simulink model "gm_IP_Core_SS_Switch_and_PWM"  (R2021a)
settings: Solver=VariableStepAuto  StartTime=0.0  StopTime=0.0002  RelTol=1e-3
undefined symbols (not defined in the file or in its folder): f_FPGA_clk, T_FPGA_clk
libraries: hdlmdlgenlib x3, hdlsllib x3
(part 2 of 2)

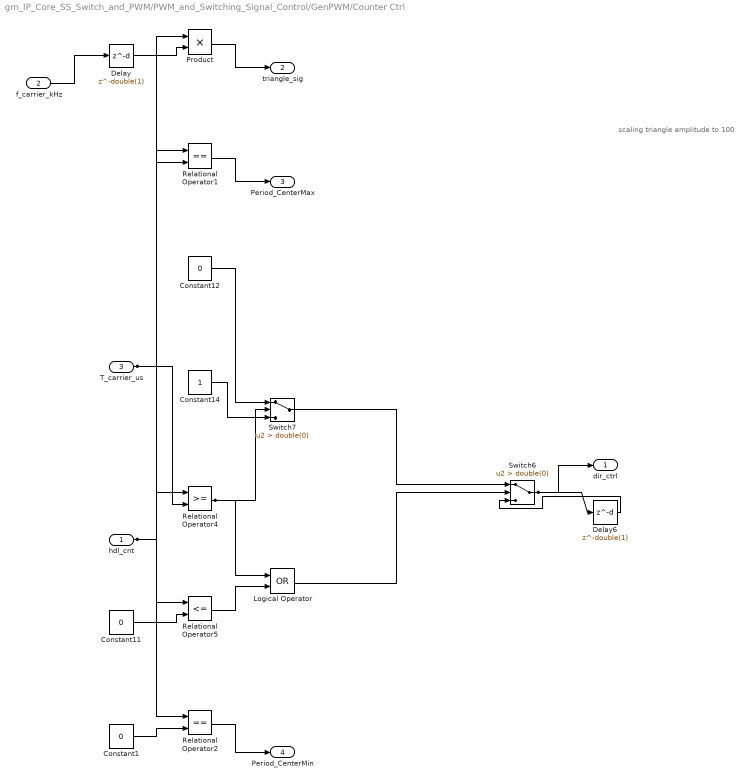
== system gm_IP_Core_SS_Switch_and_PWM/PWM_and_Switching_Signal_Control/GenPWM/Counter Ctrl ==
  note: scaling triangle amplitude to 100
  hdl_cnt : Inport  OutDataTypeStr=fixdt(0, 20, 0)  PortDimensions=1  SampleTime=1e-08
  f_carrier_kHz : Inport  Port=2  OutDataTypeStr=fixdt(0, 25, 26)  PortDimensions=1  SampleTime=1e-08
  T_carrier_us : Inport  Port=3  OutDataTypeStr=fixdt(0, 25, 0)  PortDimensions=1  SampleTime=1e-08
  Constant1 : Constant  Value=0  OutDataTypeStr=fixdt(0, 20, 0)  SampleTime=1e-08
  Constant11 : Constant  Value=0  OutDataTypeStr=fixdt(0, 20, 0)  SampleTime=1e-08
  Constant12 : Constant  Value=0  OutDataTypeStr=boolean  SampleTime=1e-08
  Constant14 : Constant  OutDataTypeStr=boolean  SampleTime=1e-08
  Delay : Delay  DelayLength=double(1)  InitialCondition=0  SampleTime=1e-08
  Delay6 : Delay  DelayLength=double(1)  InitialCondition=0  SampleTime=1e-08
  Logical Operator : Logic  Operator=OR  AllPortsSameDT=off  OutDataTypeStr=boolean  SampleTime=1e-08
  Product : Product  Inputs=**  OutDataTypeStr=fixdt(0, 18, 17)  SampleTime=1e-08
  Relational Operator1 : RelationalOperator  Operator===  OutDataTypeStr=boolean  SampleTime=1e-08  RndMeth=Nearest
  Relational Operator2 : RelationalOperator  Operator===  OutDataTypeStr=boolean  SampleTime=1e-08  RndMeth=Nearest
  Relational Operator4 : RelationalOperator  OutDataTypeStr=boolean  SampleTime=1e-08  RndMeth=Nearest
  Relational Operator5 : RelationalOperator  Operator=<=  OutDataTypeStr=boolean  SampleTime=1e-08  RndMeth=Nearest
  Switch6 : Switch  Criteria=u2 > Threshold  Threshold=double(0)  OutDataTypeStr=boolean  SampleTime=1e-08
  Switch7 : Switch  Criteria=u2 > Threshold  Threshold=double(0)  OutDataTypeStr=boolean  SampleTime=1e-08
  dir_ctrl : Outport  SampleTime=1e-08  VectorParamsAs1DForOutWhenUnconnected=off
  triangle_sig : Outport  Port=2  SampleTime=1e-08  VectorParamsAs1DForOutWhenUnconnected=off
  Period_CenterMax : Outport  Port=3  SampleTime=1e-08  VectorParamsAs1DForOutWhenUnconnected=off
  Period_CenterMin : Outport  Port=4  SampleTime=1e-08  VectorParamsAs1DForOutWhenUnconnected=off
  wires:
  hdl_cnt/1 -> Relational Operator5/1, Relational Operator4/1, Relational Operator2/1, Relational Operator1/1, Product/1
  f_carrier_kHz/1 -> Delay/1
  T_carrier_us/1 -> Relational Operator4/2, Relational Operator1/2
  Constant1/1 -> Relational Operator2/2
  Constant11/1 -> Relational Operator5/2
  Constant12/1 -> Switch7/1
  Constant14/1 -> Switch7/3
  Delay/1 -> Product/2
  Delay6/1 -> Switch6/3
  Logical Operator/1 -> Switch6/2
  Product/1 -> triangle_sig/1
  Relational Operator1/1 -> Period_CenterMax/1
  Relational Operator2/1 -> Period_CenterMin/1
  Relational Operator4/1 -> Switch7/2, Logical Operator/1
  Relational Operator5/1 -> Logical Operator/2
  Switch6/1 -> Delay6/1, dir_ctrl/1
  Switch7/1 -> Switch6/1

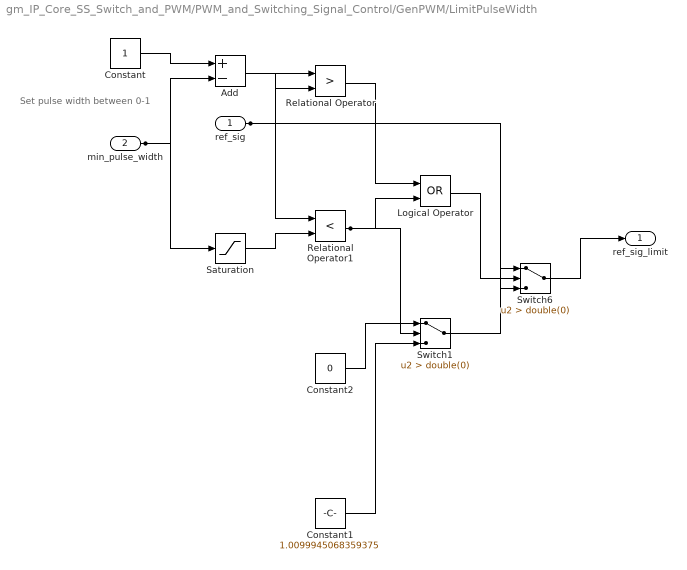
== system gm_IP_Core_SS_Switch_and_PWM/PWM_and_Switching_Signal_Control/GenPWM/LimitPulseWidth ==
  note: Set pulse width between 0-1
  ref_sig : Inport  OutDataTypeStr=fixdt(1, 14, 12)  PortDimensions=1  SampleTime=1e-08
  min_pulse_width : Inport  Port=2  OutDataTypeStr=fixdt(1, 18, 16)  PortDimensions=1  SampleTime=1e-08
  Add : Sum  Inputs=+-  AccumDataTypeStr=fixdt(1, 19, 16)  OutDataTypeStr=fixdt(1, 18, 16)  SampleTime=1e-08
  Constant : Constant  OutDataTypeStr=fixdt(1, 18, 16)  SampleTime=1e-08
  Constant1 : Constant  Value=1.0099945068359375  OutDataTypeStr=fixdt(1, 18, 16)  SampleTime=1e-08
  Constant2 : Constant  Value=0  OutDataTypeStr=fixdt(1, 18, 16)  SampleTime=1e-08
  Logical Operator : Logic  Operator=OR  AllPortsSameDT=off  OutDataTypeStr=boolean  SampleTime=1e-08
  Relational Operator : RelationalOperator  Operator=>  OutDataTypeStr=boolean  SampleTime=1e-08  RndMeth=Nearest
  Relational Operator1 : RelationalOperator  Operator=<  OutDataTypeStr=boolean  SampleTime=1e-08  RndMeth=Nearest
  Saturation : Saturate  UpperLimit="fi(0,1,18,16,\"hex\",\"10000\")"  LowerLimit="fi(0,1,18,16,\"hex\",\"00000\")"  SampleTime=1e-08  OutDataTypeStr=fixdt(1, 18, 16)
  Switch1 : Switch  Criteria=u2 > Threshold  Threshold=double(0)  OutDataTypeStr=fixdt(1, 18, 16)  SampleTime=1e-08
  Switch6 : Switch  Criteria=u2 > Threshold  Threshold=double(0)  OutDataTypeStr=fixdt(1, 18, 16)  SampleTime=1e-08
  ref_sig_limit : Outport  SampleTime=1e-08  VectorParamsAs1DForOutWhenUnconnected=off
  wires:
  Add/1 -> Relational Operator/2
  Constant/1 -> Add/1
  Constant1/1 -> Switch1/3
  Constant2/1 -> Switch1/1
  Logical Operator/1 -> Switch6/2
  Relational Operator/1 -> Logical Operator/1
  Relational Operator1/1 -> Switch1/2, Logical Operator/2
  Saturation/1 -> Relational Operator1/2
  Switch1/1 -> Switch6/1
  Switch6/1 -> ref_sig_limit/1
  ref_sig/1 -> Switch6/3, Relational Operator1/1, Relational Operator/1
  min_pulse_width/1 -> Saturation/1, Add/2

== system gm_IP_Core_SS_Switch_and_PWM/PWM_and_Switching_Signal_Control/GenPWM/LimitPulseWidth1 ==
  note: Set pulse width in percent
  ref_sig : Inport  OutDataTypeStr=fixdt(1, 14, 12)  PortDimensions=1  SampleTime=1e-08
  min_pulse_width : Inport  Port=2  OutDataTypeStr=fixdt(1, 18, 16)  PortDimensions=1  SampleTime=1e-08
  Add : Sum  Inputs=+-  AccumDataTypeStr=fixdt(1, 19, 16)  OutDataTypeStr=fixdt(1, 18, 16)  SampleTime=1e-08
  Constant : Constant  OutDataTypeStr=fixdt(1, 18, 16)  SampleTime=1e-08
  Constant1 : Constant  Value=1.0099945068359375  OutDataTypeStr=fixdt(1, 18, 16)  SampleTime=1e-08
  Constant2 : Constant  Value=0  OutDataTypeStr=fixdt(1, 18, 16)  SampleTime=1e-08
  Logical Operator : Logic  Operator=OR  AllPortsSameDT=off  OutDataTypeStr=boolean  SampleTime=1e-08
  Relational Operator : RelationalOperator  Operator=>  OutDataTypeStr=boolean  SampleTime=1e-08  RndMeth=Nearest
  Relational Operator1 : RelationalOperator  Operator=<  OutDataTypeStr=boolean  SampleTime=1e-08  RndMeth=Nearest
  Saturation : Saturate  UpperLimit="fi(0,1,18,16,\"hex\",\"10000\")"  LowerLimit="fi(0,1,18,16,\"hex\",\"00000\")"  SampleTime=1e-08  OutDataTypeStr=fixdt(1, 18, 16)
  Switch1 : Switch  Criteria=u2 > Threshold  Threshold=double(0)  OutDataTypeStr=fixdt(1, 18, 16)  SampleTime=1e-08
  Switch6 : Switch  Criteria=u2 > Threshold  Threshold=double(0)  OutDataTypeStr=fixdt(1, 18, 16)  SampleTime=1e-08
  ref_sig_limit : Outport  SampleTime=1e-08  VectorParamsAs1DForOutWhenUnconnected=off
  wires:
  Add/1 -> Relational Operator/2
  Constant/1 -> Add/1
  Constant1/1 -> Switch1/3
  Constant2/1 -> Switch1/1
  Logical Operator/1 -> Switch6/2
  Relational Operator/1 -> Logical Operator/1
  Relational Operator1/1 -> Switch1/2, Logical Operator/2
  Saturation/1 -> Relational Operator1/2
  Switch1/1 -> Switch6/1
  Switch6/1 -> ref_sig_limit/1
  ref_sig/1 -> Switch6/3, Relational Operator1/1, Relational Operator/1
  min_pulse_width/1 -> Saturation/1, Add/2

== system gm_IP_Core_SS_Switch_and_PWM/PWM_and_Switching_Signal_Control/GenPWM/LimitPulseWidth2 ==
  note: Set pulse width in percent
  ref_sig : Inport  OutDataTypeStr=fixdt(1, 14, 12)  PortDimensions=1  SampleTime=1e-08
  min_pulse_width : Inport  Port=2  OutDataTypeStr=fixdt(1, 18, 16)  PortDimensions=1  SampleTime=1e-08
  Add : Sum  Inputs=+-  AccumDataTypeStr=fixdt(1, 19, 16)  OutDataTypeStr=fixdt(1, 18, 16)  SampleTime=1e-08
  Constant : Constant  OutDataTypeStr=fixdt(1, 18, 16)  SampleTime=1e-08
  Constant1 : Constant  Value=1.0099945068359375  OutDataTypeStr=fixdt(1, 18, 16)  SampleTime=1e-08
  Constant2 : Constant  Value=0  OutDataTypeStr=fixdt(1, 18, 16)  SampleTime=1e-08
  Logical Operator : Logic  Operator=OR  AllPortsSameDT=off  OutDataTypeStr=boolean  SampleTime=1e-08
  Relational Operator : RelationalOperator  Operator=>  OutDataTypeStr=boolean  SampleTime=1e-08  RndMeth=Nearest
  Relational Operator1 : RelationalOperator  Operator=<  OutDataTypeStr=boolean  SampleTime=1e-08  RndMeth=Nearest
  Saturation : Saturate  UpperLimit="fi(0,1,18,16,\"hex\",\"10000\")"  LowerLimit="fi(0,1,18,16,\"hex\",\"00000\")"  SampleTime=1e-08  OutDataTypeStr=fixdt(1, 18, 16)
  Switch1 : Switch  Criteria=u2 > Threshold  Threshold=double(0)  OutDataTypeStr=fixdt(1, 18, 16)  SampleTime=1e-08
  Switch6 : Switch  Criteria=u2 > Threshold  Threshold=double(0)  OutDataTypeStr=fixdt(1, 18, 16)  SampleTime=1e-08
  ref_sig_limit : Outport  SampleTime=1e-08  VectorParamsAs1DForOutWhenUnconnected=off
  wires:
  Add/1 -> Relational Operator/2
  Constant/1 -> Add/1
  Constant1/1 -> Switch1/3
  Constant2/1 -> Switch1/1
  Logical Operator/1 -> Switch6/2
  Relational Operator/1 -> Logical Operator/1
  Relational Operator1/1 -> Switch1/2, Logical Operator/2
  Saturation/1 -> Relational Operator1/2
  Switch1/1 -> Switch6/1
  Switch6/1 -> ref_sig_limit/1
  ref_sig/1 -> Switch6/3, Relational Operator1/1, Relational Operator/1
  min_pulse_width/1 -> Saturation/1, Add/2

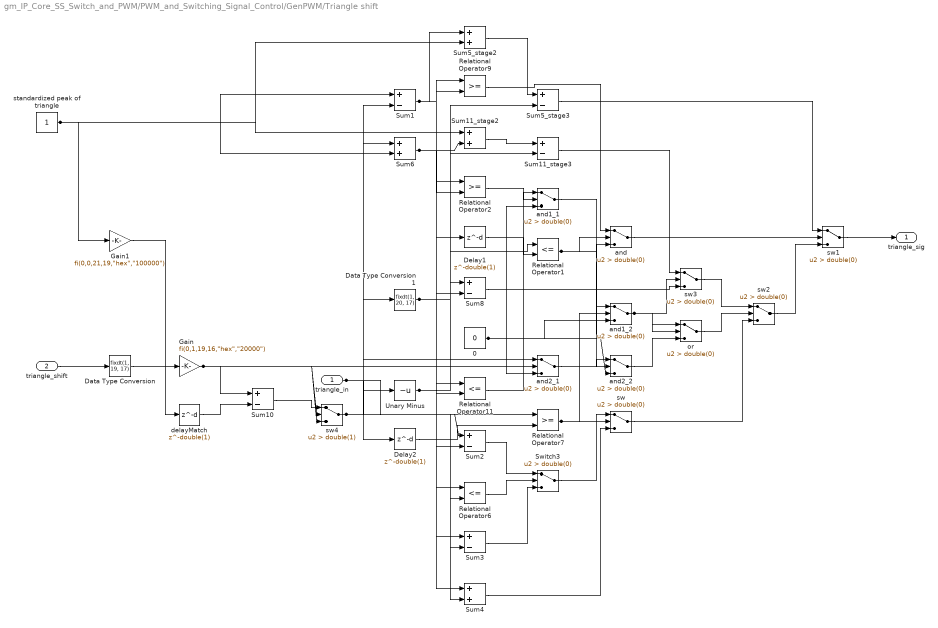
== system gm_IP_Core_SS_Switch_and_PWM/PWM_and_Switching_Signal_Control/GenPWM/Triangle shift ==
  triangle_in : Inport  OutDataTypeStr=fixdt(0, 18, 17)  PortDimensions=1  SampleTime=1e-08
  triangle_shift : Inport  Port=2  OutDataTypeStr=fixdt(0, 18, 17)  PortDimensions=1  SampleTime=1e-08
  0 : Constant  Value=0  OutDataTypeStr=boolean  SampleTime=1e-08
  Data Type Conversion : DataTypeConversion  OutDataTypeStr=fixdt(1, 19, 17)  SampleTime=1e-08
  Data Type Conversion1 : DataTypeConversion  OutDataTypeStr=fixdt(1, 20, 17)  SampleTime=1e-08
  Delay1 : Delay  DelayLength=double(1)  InitialCondition=0  SampleTime=1e-08
  Delay2 : Delay  DelayLength=double(1)  InitialCondition=0  SampleTime=1e-08
  Gain : Gain  Gain="fi(0,1,19,16,\"hex\",\"20000\")"  ParamDataTypeStr=fixdt(1, 19, 16)  OutDataTypeStr=fixdt(1, 20, 17)  SampleTime=1e-08
  Gain1 : Gain  Gain="fi(0,0,21,19,\"hex\",\"100000\")"  ParamDataTypeStr=fixdt(0, 21, 19)  OutDataTypeStr=fixdt(1, 20, 17)  SampleTime=1e-08
  Relational Operator1 : RelationalOperator  Operator=<=  OutDataTypeStr=boolean  SampleTime=1e-08  RndMeth=Nearest
  Relational Operator11 : RelationalOperator  Operator=<=  OutDataTypeStr=boolean  SampleTime=1e-08  RndMeth=Nearest
  Relational Operator2 : RelationalOperator  OutDataTypeStr=boolean  SampleTime=1e-08  RndMeth=Nearest
  Relational Operator6 : RelationalOperator  Operator=<=  OutDataTypeStr=boolean  SampleTime=1e-08  RndMeth=Nearest
  Relational Operator7 : RelationalOperator  OutDataTypeStr=boolean  SampleTime=1e-08  RndMeth=Nearest
  Relational Operator9 : RelationalOperator  OutDataTypeStr=boolean  SampleTime=1e-08  RndMeth=Nearest
  Sum1 : Sum  Inputs=+-  AccumDataTypeStr=fixdt(1, 23, 17)  OutDataTypeStr=fixdt(1, 23, 17)  SampleTime=1e-08
  Sum10 : Sum  Inputs=+-  AccumDataTypeStr=fixdt(1, 21, 17)  OutDataTypeStr=fixdt(1, 20, 17)  SampleTime=1e-08
  Sum11_stage2 : Sum  AccumDataTypeStr=fixdt(1, 24, 17)  OutDataTypeStr=fixdt(1, 24, 17)  SampleTime=1e-08
  Sum11_stage3 : Sum  Inputs=+-  AccumDataTypeStr=fixdt(1, 24, 17)  OutDataTypeStr=fixdt(1, 21, 17)  SampleTime=1e-08
  Sum2 : Sum  Inputs=+-  AccumDataTypeStr=fixdt(1, 21, 17)  OutDataTypeStr=fixdt(1, 21, 17)  SampleTime=1e-08
  Sum3 : Sum  Inputs=+-  AccumDataTypeStr=fixdt(1, 21, 17)  OutDataTypeStr=fixdt(1, 21, 17)  SampleTime=1e-08
  Sum4 : Sum  AccumDataTypeStr=fixdt(1, 21, 17)  OutDataTypeStr=fixdt(1, 21, 17)  SampleTime=1e-08
  Sum5_stage2 : Sum  AccumDataTypeStr=fixdt(1, 24, 17)  OutDataTypeStr=fixdt(1, 24, 17)  SampleTime=1e-08
  Sum5_stage3 : Sum  Inputs=+-  AccumDataTypeStr=fixdt(1, 24, 17)  OutDataTypeStr=fixdt(1, 21, 17)  SampleTime=1e-08
  Sum6 : Sum  AccumDataTypeStr=fixdt(1, 23, 17)  OutDataTypeStr=fixdt(1, 23, 17)  SampleTime=1e-08
  Sum8 : Sum  Inputs=+-  AccumDataTypeStr=fixdt(1, 21, 17)  OutDataTypeStr=fixdt(1, 21, 17)  SampleTime=1e-08
  Switch3 : Switch  Criteria=u2 > Threshold  Threshold=double(0)  OutDataTypeStr=fixdt(1, 21, 17)  SampleTime=1e-08
  Unary Minus : UnaryMinus  SampleTime=1e-08
  and : Switch  Criteria=u2 > Threshold  Threshold=double(0)  OutDataTypeStr=boolean  SampleTime=1e-08
  and1_1 : Switch  Criteria=u2 > Threshold  Threshold=double(0)  OutDataTypeStr=boolean  SampleTime=1e-08
  and1_2 : Switch  Criteria=u2 > Threshold  Threshold=double(0)  OutDataTypeStr=boolean  SampleTime=1e-08
  and2_1 : Switch  Criteria=u2 > Threshold  Threshold=double(0)  OutDataTypeStr=boolean  SampleTime=1e-08
  and2_2 : Switch  Criteria=u2 > Threshold  Threshold=double(0)  OutDataTypeStr=boolean  SampleTime=1e-08
  delayMatch : Delay  DelayLength=double(1)  InitialCondition=0  SampleTime=1e-08
  or : Switch  Criteria=u2 > Threshold  Threshold=double(0)  OutDataTypeStr=boolean  SampleTime=1e-08
  standardized peak of triangle : Constant  OutDataTypeStr=fixdt(0, 21, 17)  SampleTime=1e-08
  sw : Switch  Criteria=u2 > Threshold  Threshold=double(0)  OutDataTypeStr=fixdt(1, 21, 17)  SampleTime=1e-08
  sw1 : Switch  Criteria=u2 > Threshold  Threshold=double(0)  OutDataTypeStr=fixdt(1, 18, 16)  SampleTime=1e-08
  sw2 : Switch  Criteria=u2 > Threshold  Threshold=double(0)  OutDataTypeStr=fixdt(1, 21, 17)  SampleTime=1e-08
  sw3 : Switch  Criteria=u2 > Threshold  Threshold=double(0)  OutDataTypeStr=fixdt(1, 21, 17)  SampleTime=1e-08
  sw4 : Switch  Criteria=u2 > Threshold  Threshold=double(1)  OutDataTypeStr=fixdt(1, 20, 17)  SampleTime=1e-08
  triangle_sig : Outport  SampleTime=1e-08  VectorParamsAs1DForOutWhenUnconnected=off
  wires:
  0/1 -> and2_2/3, and2_1/3, and1_2/3, and1_1/3, and/3
  Data Type Conversion/1 -> Gain/1
  Data Type Conversion1/1 -> Sum8/2, Sum5_stage3/2, Sum4/1, Sum3/1, Sum2/2, Sum11_stage3/2, Relational Operator9/1, Relational Operator6/1, Relational Operator2/1, Relational Operator11/1, Relational Operator1/1, Delay1/1
  Delay1/1 -> Relational Operator1/2
  Delay2/1 -> Relational Operator7/2
  Gain/1 -> sw4/3, sw4/2, and2_1/1, and1_1/1, Sum10/1
  delayMatch/1 -> Sum10/2
  Relational Operator1/1 -> and2_2/2, and/2
  Relational Operator11/1 -> and2_1/2
  Relational Operator2/1 -> and1_1/2
  Relational Operator6/1 -> Switch3/2
  Relational Operator7/1 -> sw/2, and1_2/2
  Relational Operator9/1 -> and/1
  Sum1/1 -> Sum5_stage2/1, Relational Operator9/2
  Sum10/1 -> sw4/1
  Sum11_stage3/1 -> sw3/1
  Sum2/1 -> Switch3/1
  Sum3/1 -> Switch3/3
  Sum4/1 -> sw/3
  Sum5_stage3/1 -> sw1/1
  Sum6/1 -> Sum11_stage2/2, Relational Operator2/2
  Sum8/1 -> sw3/3
  Switch3/1 -> sw/1
  Unary Minus/1 -> Sum8/1, Relational Operator11/2
  and/1 -> sw1/2
  and1_1/1 -> and1_2/1
  and1_2/1 -> sw3/2, or/2, or/1
  and2_1/1 -> and2_2/1
  and2_2/1 -> or/3
  or/1 -> sw2/2
  standardized peak of triangle/1 -> Sum6/2, Sum5_stage2/2, Sum11_stage2/1, Sum1/1, Gain1/1
  sw/1 -> sw2/3
  sw1/1 -> triangle_sig/1
  sw2/1 -> sw1/3
  sw3/1 -> sw2/1
  sw4/1 -> Unary Minus/1, Sum6/1, Sum4/2, Sum3/2, Sum2/1, Sum1/2, Relational Operator6/2
  Sum11_stage2/1 -> Sum11_stage3/1
  Sum5_stage2/1 -> Sum5_stage3/1
  triangle_in/1 -> Relational Operator7/1, Data Type Conversion1/1, Delay2/1
  triangle_shift/1 -> Data Type Conversion/1
  Gain1/1 -> delayMatch/1

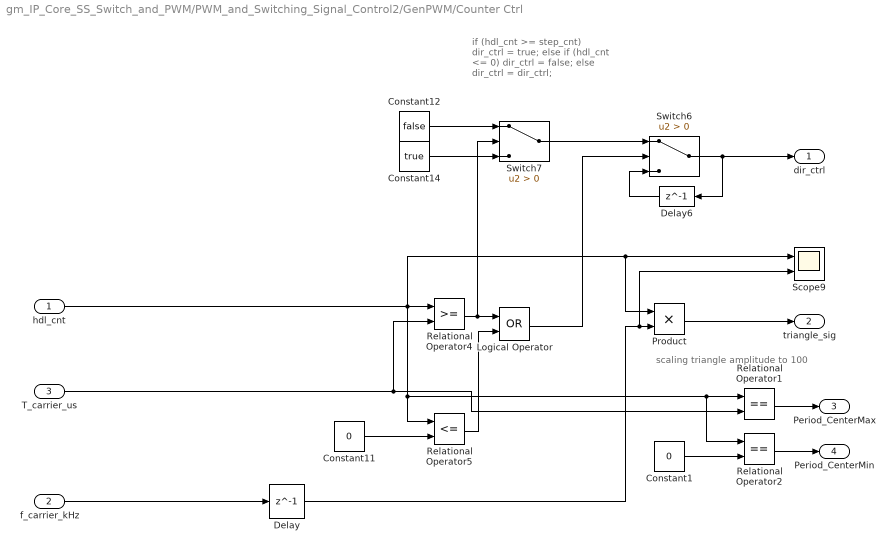
== system gm_IP_Core_SS_Switch_and_PWM/PWM_and_Switching_Signal_Control2/GenPWM/Counter Ctrl ==
  note: scaling triangle amplitude to 100
  note: if (hdl_cnt >= step_cnt)
      | 	dir_ctrl = true;
      | else if (hdl_cnt <= 0)
      | 	dir_ctrl = false;
      | else
      | 	dir_ctrl = dir_ctrl;
  hdl_cnt : Inport
  f_carrier_kHz : Inport  Port=2
  T_carrier_us : Inport  Port=3
  Constant1 : Constant  Value=0  OutDataTypeStr=fixdt(0,20,0)  SampleTime=T_FPGA_clk
  Constant11 : Constant  Value=0  OutDataTypeStr=fixdt(0,20,0)  SampleTime=T_FPGA_clk
  Constant12 : Constant  Value=false  SampleTime=T_FPGA_clk
  Constant14 : Constant  Value=true  SampleTime=T_FPGA_clk
  Delay : Delay  DelayLength=1
  Delay6 : Delay  DelayLength=1
  Logical Operator : Logic  Operator=OR  AllPortsSameDT=off  OutDataTypeStr=boolean
  Product : Product  OutDataTypeStr=fixdt(0,18,17)
  Relational Operator1 : RelationalOperator  Operator===  OutDataTypeStr=boolean  RndMeth=Nearest
  Relational Operator2 : RelationalOperator  Operator===  OutDataTypeStr=boolean  RndMeth=Nearest
  Relational Operator4 : RelationalOperator  OutDataTypeStr=boolean  RndMeth=Nearest
  Relational Operator5 : RelationalOperator  Operator=<=  OutDataTypeStr=boolean  RndMeth=Nearest
  Scope9 : Scope  NumInputPorts=2
  Switch6 : Switch  Criteria=u2 > Threshold
  Switch7 : Switch  Criteria=u2 > Threshold
  dir_ctrl : Outport  VectorParamsAs1DForOutWhenUnconnected=off
  triangle_sig : Outport  Port=2  VectorParamsAs1DForOutWhenUnconnected=off
  Period_CenterMax : Outport  Port=3  VectorParamsAs1DForOutWhenUnconnected=off
  Period_CenterMin : Outport  Port=4  VectorParamsAs1DForOutWhenUnconnected=off
  wires:
  Product/1 -> triangle_sig/1
  Constant1/1 -> Relational Operator2/2
  Relational Operator2/1 -> Period_CenterMin/1
  Relational Operator1/1 -> Period_CenterMax/1
  Delay/1 -> Product/2, Scope9/2
  f_carrier_kHz/1 -> Delay/1
  T_carrier_us/1 -> Relational Operator1/2, Relational Operator4/2
  Delay6/1 -> Switch6/3
  Constant14/1 -> Switch7/3
  Constant12/1 -> Switch7/1
  Switch7/1 -> Switch6/1
  Logical Operator/1 -> Switch6/2
  Constant11/1 -> Relational Operator5/2
  Relational Operator5/1 -> Logical Operator/2
  Relational Operator4/1 -> Logical Operator/1, Switch7/2
  Switch6/1 -> dir_ctrl/1, Delay6/1
  hdl_cnt/1 -> Scope9/1, Product/1, Relational Operator4/1, Relational Operator5/1, Relational Operator1/1, Relational Operator2/1

== system gm_IP_Core_SS_Switch_and_PWM/PWM_and_Switching_Signal_Control2/GenPWM/LimitPulseWidth ==
  note: Set pulse width between 0-1
  ref_sig : Inport
  min_pulse_width : Inport  Port=2
  Add : Sum  Inputs=+-  OutDataTypeStr=Inherit: Same as first input
  Constant : Constant  OutDataTypeStr=fixdt(1,18,16)  SampleTime=T_FPGA_clk
  Constant1 : Constant  Value=1.01  OutDataTypeStr=fixdt(1,18,16)  SampleTime=T_FPGA_clk
  Constant2 : Constant  Value=0  OutDataTypeStr=fixdt(1,18,16)  SampleTime=T_FPGA_clk
  Logical Operator : Logic  Operator=OR  AllPortsSameDT=off  OutDataTypeStr=boolean
  Relational Operator : RelationalOperator  Operator=>  OutDataTypeStr=boolean  RndMeth=Nearest
  Relational Operator1 : RelationalOperator  Operator=<  OutDataTypeStr=boolean  RndMeth=Nearest
  Saturation : Saturate  UpperLimit=1  LowerLimit=0  OutDataTypeStr=fixdt(1,18,16)
  Switch1 : Switch  Criteria=u2 > Threshold
  Switch6 : Switch  Criteria=u2 > Threshold
  ref_sig_limit : Outport  VectorParamsAs1DForOutWhenUnconnected=off
  wires:
  Saturation/1 -> Relational Operator1/2
  Switch6/1 -> ref_sig_limit/1
  Constant2/1 -> Switch1/1
  Switch1/1 -> Switch6/1
  Constant1/1 -> Switch1/3
  Logical Operator/1 -> Switch6/2
  Relational Operator1/1 -> Switch1/2, Logical Operator/2
  Relational Operator/1 -> Logical Operator/1
  ref_sig/1 -> Relational Operator1/1, Relational Operator/1, Switch6/3
  Add/1 -> Relational Operator/2
  min_pulse_width/1 -> Saturation/1, Add/2
  Constant/1 -> Add/1

== system gm_IP_Core_SS_Switch_and_PWM/PWM_and_Switching_Signal_Control2/GenPWM/LimitPulseWidth1 ==
  note: Set pulse width in percent
  ref_sig : Inport
  min_pulse_width : Inport  Port=2
  Add : Sum  Inputs=+-  OutDataTypeStr=Inherit: Same as first input
  Constant : Constant  OutDataTypeStr=fixdt(1,18,16)  SampleTime=T_FPGA_clk
  Constant1 : Constant  Value=1.01  OutDataTypeStr=fixdt(1,18,16)  SampleTime=T_FPGA_clk
  Constant2 : Constant  Value=0  OutDataTypeStr=fixdt(1,18,16)  SampleTime=T_FPGA_clk
  Logical Operator : Logic  Operator=OR  AllPortsSameDT=off  OutDataTypeStr=boolean
  Relational Operator : RelationalOperator  Operator=>  OutDataTypeStr=boolean  RndMeth=Nearest
  Relational Operator1 : RelationalOperator  Operator=<  OutDataTypeStr=boolean  RndMeth=Nearest
  Saturation : Saturate  UpperLimit=1  LowerLimit=0  OutDataTypeStr=fixdt(1,18,16)
  Switch1 : Switch  Criteria=u2 > Threshold
  Switch6 : Switch  Criteria=u2 > Threshold
  ref_sig_limit : Outport  VectorParamsAs1DForOutWhenUnconnected=off
  wires:
  Saturation/1 -> Relational Operator1/2
  Switch6/1 -> ref_sig_limit/1
  Constant2/1 -> Switch1/1
  Switch1/1 -> Switch6/1
  Constant1/1 -> Switch1/3
  Logical Operator/1 -> Switch6/2
  Relational Operator1/1 -> Switch1/2, Logical Operator/2
  Relational Operator/1 -> Logical Operator/1
  ref_sig/1 -> Relational Operator1/1, Relational Operator/1, Switch6/3
  Add/1 -> Relational Operator/2
  min_pulse_width/1 -> Saturation/1, Add/2
  Constant/1 -> Add/1

== system gm_IP_Core_SS_Switch_and_PWM/PWM_and_Switching_Signal_Control2/GenPWM/LimitPulseWidth2 ==
  note: Set pulse width in percent
  ref_sig : Inport
  min_pulse_width : Inport  Port=2
  Add : Sum  Inputs=+-  OutDataTypeStr=Inherit: Same as first input
  Constant : Constant  OutDataTypeStr=fixdt(1,18,16)  SampleTime=T_FPGA_clk
  Constant1 : Constant  Value=1.01  OutDataTypeStr=fixdt(1,18,16)  SampleTime=T_FPGA_clk
  Constant2 : Constant  Value=0  OutDataTypeStr=fixdt(1,18,16)  SampleTime=T_FPGA_clk
  Logical Operator : Logic  Operator=OR  AllPortsSameDT=off  OutDataTypeStr=boolean
  Relational Operator : RelationalOperator  Operator=>  OutDataTypeStr=boolean  RndMeth=Nearest
  Relational Operator1 : RelationalOperator  Operator=<  OutDataTypeStr=boolean  RndMeth=Nearest
  Saturation : Saturate  UpperLimit=1  LowerLimit=0  OutDataTypeStr=fixdt(1,18,16)
  Switch1 : Switch  Criteria=u2 > Threshold
  Switch6 : Switch  Criteria=u2 > Threshold
  ref_sig_limit : Outport  VectorParamsAs1DForOutWhenUnconnected=off
  wires:
  Saturation/1 -> Relational Operator1/2
  Switch6/1 -> ref_sig_limit/1
  Constant2/1 -> Switch1/1
  Switch1/1 -> Switch6/1
  Constant1/1 -> Switch1/3
  Logical Operator/1 -> Switch6/2
  Relational Operator1/1 -> Switch1/2, Logical Operator/2
  Relational Operator/1 -> Logical Operator/1
  ref_sig/1 -> Relational Operator1/1, Relational Operator/1, Switch6/3
  Add/1 -> Relational Operator/2
  min_pulse_width/1 -> Saturation/1, Add/2
  Constant/1 -> Add/1

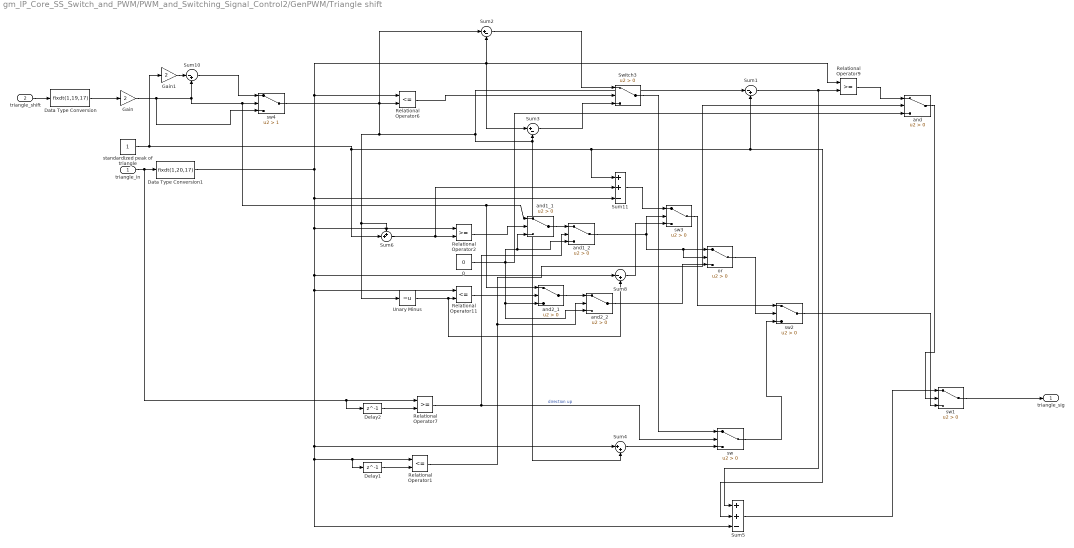
== system gm_IP_Core_SS_Switch_and_PWM/PWM_and_Switching_Signal_Control2/GenPWM/Triangle shift ==
  triangle_in : Inport
  triangle_shift : Inport  Port=2
  0 : Constant  Value=0  OutDataTypeStr=boolean  SampleTime=T_FPGA_clk
  Data Type Conversion : DataTypeConversion  OutDataTypeStr=fixdt(1,19,17)
  Data Type Conversion1 : DataTypeConversion  OutDataTypeStr=fixdt(1,20,17)
  Delay1 : Delay  DelayLength=1
  Delay2 : Delay  DelayLength=1
  Gain : Gain  Gain=2  OutDataTypeStr=fixdt(1,20,17)
  Gain1 : Gain  Gain=2  OutDataTypeStr=fixdt(1,20,17)
  Relational Operator1 : RelationalOperator  Operator=<=  OutDataTypeStr=boolean  RndMeth=Nearest
  Relational Operator11 : RelationalOperator  Operator=<=  OutDataTypeStr=boolean  RndMeth=Nearest
  Relational Operator2 : RelationalOperator  OutDataTypeStr=boolean  RndMeth=Nearest
  Relational Operator6 : RelationalOperator  Operator=<=  OutDataTypeStr=boolean  RndMeth=Nearest
  Relational Operator7 : RelationalOperator  OutDataTypeStr=boolean  RndMeth=Nearest
  Relational Operator9 : RelationalOperator  OutDataTypeStr=boolean  RndMeth=Nearest
  Sum1 : Sum  Inputs=|-+
  Sum10 : Sum  Inputs=|-+  OutDataTypeStr=fixdt(1,20,17)
  Sum11 : Sum  Inputs=++-  OutDataTypeStr=fixdt(1,21,17)
  Sum2 : Sum  Inputs=|+-
  Sum3 : Sum  Inputs=|+-
  Sum4 : Sum  Inputs=|++
  Sum5 : Sum  Inputs=++-  OutDataTypeStr=fixdt(1,21,17)
  Sum6 : Sum  Inputs=++|
  Sum8 : Sum  Inputs=|-+
  Switch3 : Switch  Criteria=u2 > Threshold
  Unary Minus : UnaryMinus
  and : Switch  Criteria=u2 > Threshold
  and1_1 : Switch  Criteria=u2 > Threshold
  and1_2 : Switch  Criteria=u2 > Threshold
  and2_1 : Switch  Criteria=u2 > Threshold
  and2_2 : Switch  Criteria=u2 > Threshold
  or : Switch  Criteria=u2 > Threshold
  standardized peak of triangle : Constant  OutDataTypeStr=fixdt(0,21,17)  SampleTime=T_FPGA_clk
  sw : Switch  Criteria=u2 > Threshold
  sw1 : Switch  Criteria=u2 > Threshold  OutDataTypeStr=fixdt(1,18,16)
  sw2 : Switch  Criteria=u2 > Threshold
  sw3 : Switch  Criteria=u2 > Threshold
  sw4 : Switch  Criteria=u2 > Threshold  Threshold=1  OutDataTypeStr=fixdt(1,20,17)
  triangle_sig : Outport  VectorParamsAs1DForOutWhenUnconnected=off
  wires:
  and2_1/1 -> and2_2/1
  0/1 -> and2_2/3, and2_1/3, and1_2/3, and1_1/3, and/3
  and1_1/1 -> and1_2/1
  Sum11/1 -> sw3/1
  and2_2/1 -> or/3
  Delay1/1 -> Relational Operator1/2
  Relational Operator1/1 -> and2_2/2, and/2
  triangle_in/1 -> Data Type Conversion1/1, Relational Operator7/1, Delay2/1
  sw/1 -> sw2/3
  Data Type Conversion/1 -> Gain/1
  and1_2/1 -> sw3/2, or/1, or/2
  sw2/1 -> sw1/3
  Gain1/1 -> Sum10/1
  triangle_shift/1 -> Data Type Conversion/1
  standardized peak of triangle/1 -> Gain1/1, Sum6/2, Sum5/2, Sum1/2, Sum11/1
  sw1/1 -> triangle_sig/1
  Sum10/1 -> sw4/1
  Gain/1 -> sw4/3, Sum10/2, sw4/2, and1_1/1, and2_1/1
  sw4/1 -> Unary Minus/1, Sum6/1, Sum1/1, Sum3/2, Sum4/2, Relational Operator6/2, Sum2/1
  or/1 -> sw2/2
  Sum2/1 -> Switch3/1
  Relational Operator9/1 -> and/1
  Sum8/1 -> sw3/3
  Sum4/1 -> sw/3
  Sum5/1 -> sw1/1
  and/1 -> sw1/2
  Sum6/1 -> Relational Operator2/2, Sum11/2
  Switch3/1 -> sw/1
  Relational Operator11/1 -> and2_1/2
  Relational Operator7/1 -> sw/2, and1_2/2  "direction up"
  Relational Operator6/1 -> Switch3/2
  sw3/1 -> sw2/1
  Unary Minus/1 -> Relational Operator11/2, Sum8/2
  Sum3/1 -> Switch3/3
  Relational Operator2/1 -> and1_1/2
  Data Type Conversion1/1 -> Relational Operator6/1, Relational Operator9/1, Sum3/1, Sum2/2, Sum11/3, Relational Operator2/1, Sum8/1, Relational Operator11/1, Sum4/1, Sum5/3, Relational Operator1/1, Delay1/1
  Delay2/1 -> Relational Operator7/2
  Sum1/1 -> Sum5/1, Relational Operator9/2
